simulink model "Ejer2_EcVanDerPol"  (R2023b)
settings: Solver=VariableStepAuto  StartTime=0  StopTime=20  RelTol=1e-3
values from neighbouring files (symbols this model uses):
  dx0 = 0    [EjerciciosModelosContinuos.m]
  mu = [5, 0, 0.3]    [EjerciciosModelosContinuos.m]
  x0 = 0    [EjerciciosModelosContinuos.m]
settings Model: Creator=alfre  LastModifiedBy=alfre

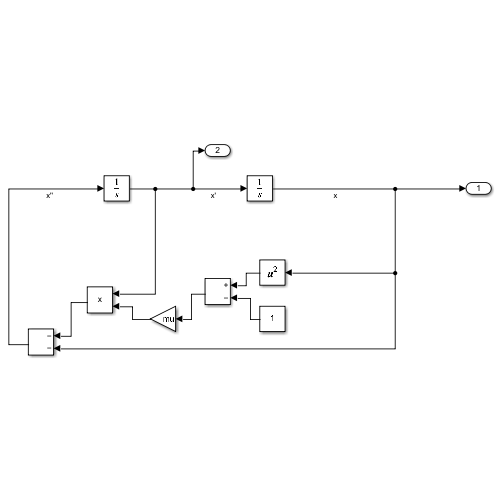
[thumbnail: Simulink's stored preview of the top-level diagram]
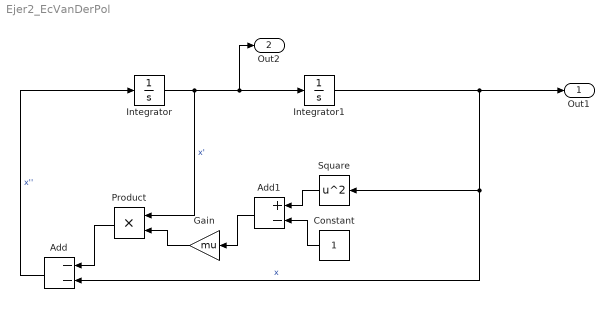
== system Ejer2_EcVanDerPol ==
  Add : Sum  Inputs=--
  Add1 : Sum  Inputs=+-
  Constant : Constant
  Gain : Gain  Gain=mu
  Integrator : Integrator  InitialCondition=dx0
  Integrator1 : Integrator  InitialCondition=x0
  Product : Product
  Square : Math  Operator=square
  Out1 : Outport
  Out2 : Outport  Port=2
  wires:
  Integrator1/1 -> Out1/1, Square/1, Add/2  "x"
  Integrator/1 -> Product/1, Out2/1, Integrator1/1  "x'"
  Square/1 -> Add1/1
  Constant/1 -> Add1/2
  Add/1 -> Integrator/1  "x''"
  Product/1 -> Add/1
  Add1/1 -> Gain/1
  Gain/1 -> Product/2
